simulink model "Target_Control_System"  (R2021b)
settings: Solver=FixedStepDiscrete  StartTime=0.0  StopTime=5  RelTol=1e-3
PreLoadFcn:
  | RTWConfigurationCB('preloadfcn', bdroot);
PostLoadFcn:
  | load('configuration/data_struct.mat');
  | load('configuration/fluxMaps_propMotor.mat');
  | load('configuration/parameterInit_PROP.mat');
  | load('configuration/parameterInit_PUMP.mat');
  | load('configuration/parameterInit_PITCH.mat');
  | load('configuration/parameterInit_TILT.mat');
  | %load('configuration/base_workspace_signal_definition.mat');
  | %load('resolvedatastores_to_baseworkspace_for_faster_simulation.mat');
model workspace (MAT data in the model file):
  SIMULATION_OPTIONS : Simulink.Parameter (value not decoded)
  TARGET_CODE_GEN : Simulink.Parameter (value not decoded)
  TCS_SAMPLE_FREQ_HZ : Simulink.Parameter (value not decoded)
symbols that are objects in the model workspace (value not decoded): TARGET_CODE_GEN, TCS_SAMPLE_FREQ_HZ
undefined symbols (not defined in the file): A_DQ_REF_LPF_INIT__PITCH, A_DQ_REF_LPF_INIT__PROP, A_DQ_REF_LPF_INIT__PUMP, A_DQ_REF_LPF_INIT__TILT, A_OBSERVER_CONFIDENCE_INIT__PITCH, A_OBSERVER_CONFIDENCE_INIT__PROP, A_OBSERVER_CONFIDENCE_INIT__PUMP, A_OBSERVER_CONFIDENCE_INIT__TILT, ACTUATOR_MAX_ANGLE_TRIP__PITCH, ACTUATOR_MIN_ANGLE_TRIP__PITCH, ACTUATOR_POS_SENSOR_INV_DIRECTION__PITCH, ACTUATOR_POS_SENSOR_INV_DIRECTION__TILT, ACTUATOR_POS_SENSOR_OFFSET__PITCH, ACTUATOR_POS_SENSOR_OFFSET__TILT, ADC_scaler1_baseaddr_TILT, ADC_SCALER_FLOAT_TO_FIXPOINT_EXPANSION, ANGLE_ELEC_FROM_SENSOR_OFFSET_INIT__PITCH, ANGLE_ELEC_FROM_SENSOR_OFFSET_INIT__PROP, ANGLE_ELEC_FROM_SENSOR_OFFSET_INIT__PUMP, ANGLE_ELEC_FROM_SENSOR_OFFSET_INIT__TILT, AUTO_CLEAR_FAULTS_ENABLED__PITCH, AUTO_CLEAR_FAULTS_ENABLED__PROP, AUTO_CLEAR_FAULTS_ENABLED__PUMP, AUTO_CLEAR_FAULTS_ENABLED__TILT, AUTO_CLEAR_FAULTS_WAIT_TICKS__PITCH, AUTO_CLEAR_FAULTS_WAIT_TICKS__PROP, AUTO_CLEAR_FAULTS_WAIT_TICKS__PUMP, AUTO_CLEAR_FAULTS_WAIT_TICKS__TILT, AUTO_I_ZERO_IDLE_TICKS__PITCH, AUTO_I_ZERO_IDLE_TICKS__PROP, AUTO_I_ZERO_IDLE_TICKS__PUMP, AUTO_I_ZERO_IDLE_TICKS__TILT, AUTO_I_ZERO_OFFSET_IDC_THRESHOLD__PITCH, AUTO_I_ZERO_OFFSET_IDC_THRESHOLD__PROP, AUTO_I_ZERO_OFFSET_IDC_THRESHOLD__PUMP, AUTO_I_ZERO_OFFSET_IDC_THRESHOLD__TILT, AUTO_I_ZERO_OFFSET_IPH_THRESHOLD__PITCH, AUTO_I_ZERO_OFFSET_IPH_THRESHOLD__PROP, AUTO_I_ZERO_OFFSET_IPH_THRESHOLD__PUMP, AUTO_I_ZERO_OFFSET_IPH_THRESHOLD__TILT, AUTO_SENSORLESS_SWITCHOVER_DISABLE_OMEGA, AUTO_SENSORLESS_SWITCHOVER_ENABLE_OMEGA, AUTO_SENSORLESS_SWITCHOVER_MIN_CONFIDENCE, AUXILIARY_PROTECTION_UNIT_BASEADDR__TILT, blanking_max_error_omega_INIT_PITCH, blanking_max_error_omega_INIT_TILT, blanking_max_error_position_INIT_PITCH, blanking_max_error_position_INIT_TILT, BRUTE_START_I_Q_REF_RAMP_SPEED__PITCH, BRUTE_START_I_Q_REF_RAMP_SPEED__PROP, BRUTE_START_I_Q_REF_RAMP_SPEED__PUMP, BRUTE_START_I_Q_REF_RAMP_SPEED__TILT, CONTROL_LOOP_DT_INIT__PITCH, CONTROL_LOOP_DT_INIT__PROP, CONTROL_LOOP_DT_INIT__PUMP, CONTROL_LOOP_DT_INIT__TILT, CORRECTION_FILTER_SCALE__PITCH, CORRECTION_FILTER_SCALE__PROP, CORRECTION_FILTER_SCALE__PUMP, CORRECTION_FILTER_SCALE__TILT ... (+458)
libraries: simulink x178, Reusables_Lib x24
(part 30 of 47)

== system Target_Control_System/Target_Control_System/MainLoop/tiltMotor_mainLoop/mainTask_tilt/motorTaskMainFastStep(&oTilt)/Control Loops - Tilt ==
  note: // Ramp Id, also include a fixed fraction of Iq (happens in the interupt)
  note: // Feed-forward of speed reference derivative into torque
      | // --- Would go here if needed --- (Blend the ramp generator ddt output into Iq ref)
  note: // Static current limiting only
  note: // The greater than 0 is needed to allow regen braking when the speed is high enough
  note: // Ramp position setpoint
  note: // Blend in the idle controller's contribution (don't add; disturbs Torque/Amp relation).
      | // Take the max of both, but only if the idle controller is active)
  note: // Ramp angle compensation value for smoothing of forced to closed loop operation
      |  // It always ramps to zero.
  note: // no feedforward in forced angle, because the speed estimate may be garbage
  controlLoops : TriggerPort  TriggerType=function-call  VariantControl=Variant
  AND1 : Logic  AllPortsSameDT=off  OutDataTypeStr=boolean
  Constant13 : Constant  Value=CONTROL_LOOP_DT_INIT__TILT  OutDataTypeStr=single  SampleTime=-1
  Constant2 : Constant  Commented=on  Value=0  SampleTime=-1
  Constant3 : Constant  Value=0  SampleTime=-1
  Constant4 : Constant  Value=0.001  OutDataTypeStr=single  SampleTime=-1
  Constant5 : Constant  Commented=on  Value=0  OutDataTypeStr=single  SampleTime=-1
  Constant6 : Constant  Value=0  OutDataTypeStr=single  SampleTime=-1
  Constant7 : Constant  Value=ISR_FREQ_KHZ__TILT  OutDataTypeStr=single  SampleTime=-1
  Data Store Read10 : DataStoreRead  DataStoreName=oTilt  DataStoreElements=oTilt.oMot_.oState_.oRampDataIdRef_.oParam_.fDownslope_  IndexOptions=Index vector (dialog)  Indices=1  OutputSizes=1
  Data Store Read104 : DataStoreRead  Commented=on  DataStoreName=oTilt  DataStoreElements=oTilt.oMot_.oOut_.uiForcedAngle_  IndexOptions=Index vector (dialog)  Indices=1  OutputSizes=1
  Data Store Read11 : DataStoreRead  DataStoreName=oTilt  DataStoreElements=oTilt.oMot_.oState_.oRampDataIdRef_.oParam_.fUpslope_  IndexOptions=Index vector (dialog)  Indices=1  OutputSizes=1
  Data Store Read110 : DataStoreRead  Commented=on  DataStoreName=oTilt  DataStoreElements=oTilt.oMot_.oState_.oRampDataFluxMstrAngFrcd2clsdSmoothn_.oParam_.fUpslope_  IndexOptions=Index vector (dialog)  Indices=1  OutputSizes=1
  Data Store Read111 : DataStoreRead  Commented=on  DataStoreName=oTilt  DataStoreElements=oTilt.oMot_.oState_.oRampDataFluxMstrAngFrcd2clsdSmoothn_.oParam_.fDownslope_  IndexOptions=Index vector (dialog)  Indices=1  OutputSizes=1
  Data Store Read112 : DataStoreRead  Commented=on  DataStoreName=oTilt  DataStoreElements=oTilt.oMot_.oState_.oRampDataFluxMstrAngFrcd2clsdSmoothn_.oParam_.fTimestepS_  IndexOptions=Index vector (dialog)  Indices=1  OutputSizes=1
  Data Store Read12 : DataStoreRead  DataStoreName=oTilt  DataStoreElements=oTilt.oMot_.oState_.oRampDataIdRef_.oParam_.fTimestepS_  IndexOptions=Index vector (dialog)  Indices=1  OutputSizes=1
  Data Store Read13 : DataStoreRead  DataStoreName=oTilt  DataStoreElements=oTilt.oMot_.oState_.oPosSensor_.iPosControlEnabled_  IndexOptions=Index vector (dialog)  Indices=1  OutputSizes=1
  Data Store Read14 : DataStoreRead  DataStoreName=oTilt  DataStoreElements=oTilt.oMot_.oState_.oRampDataOmegaERef_.fSetpoint_  IndexOptions=Index vector (dialog)  Indices=1  OutputSizes=1
  Data Store Read15 : DataStoreRead  DataStoreName=oTilt  DataStoreElements=oTilt.oMot_.oParam_.fDynILimIntegratorLeakageFactor_  IndexOptions=Index vector (dialog)  Indices=1  OutputSizes=1
  Data Store Read16 : DataStoreRead  DataStoreName=oTilt  DataStoreElements=oTilt.oMot_.oState_.fIdleCtrlCurrent_  IndexOptions=Index vector (dialog)  Indices=1  OutputSizes=1
  Data Store Read17 : DataStoreRead  DataStoreName=oTilt  DataStoreElements=oTilt.oMot_.oParam_.fIqSetpointMax_  IndexOptions=Index vector (dialog)  Indices=1  OutputSizes=1
  Data Store Read19 : DataStoreRead  DataStoreName=oTilt  DataStoreElements=oTilt.oMot_.oParam_.fPositionRefFfwdToOmega_  IndexOptions=Index vector (dialog)  Indices=1  OutputSizes=1
  Data Store Read2 : DataStoreRead  Commented=on  DataStoreName=oTilt  DataStoreElements=oTilt.oMot_.oState_.oRampDataFluxMasterAngleOffset_.fSetpoint_  IndexOptions=Index vector (dialog)  Indices=1  OutputSizes=1
  Data Store Read20 : DataStoreRead  DataStoreName=oTilt  DataStoreElements=oTilt.oMot_.oState_.oRampDataIqRef_.oParam_.fUpslope_  IndexOptions=Index vector (dialog)  Indices=1  OutputSizes=1
  Data Store Read21 : DataStoreRead  DataStoreName=oTilt  DataStoreElements=oTilt.oMot_.oState_.fIqRefBeforeRamp_  IndexOptions=Index vector (dialog)  Indices=1  OutputSizes=1
  Data Store Read22 : DataStoreRead  DataStoreName=oTilt  DataStoreElements=oTilt.oMot_.oState_.oRampDataIqRef_.oParam_.fDownslope_  IndexOptions=Index vector (dialog)  Indices=1  OutputSizes=1
  Data Store Read23 : DataStoreRead  Commented=on  DataStoreName=oTilt  DataStoreElements=oTilt.oMot_.oState_.oRampDataFluxFeedforwardGain_.fRampOut_  IndexOptions=Index vector (dialog)  Indices=1  OutputSizes=1
  Data Store Read27 : DataStoreRead  DataStoreName=oTilt  DataStoreElements=oTilt.oMot_.oState_.oRampDataOmegaERef_.oParam_.fUpslope_  IndexOptions=Index vector (dialog)  Indices=1  OutputSizes=1
  Data Store Read28 : DataStoreRead  DataStoreName=oTilt  DataStoreElements=oTilt.oMot_.oState_.uiSpeedControllerActive_  IndexOptions=Index vector (dialog)  Indices=1  OutputSizes=1
  Data Store Read29 : DataStoreRead  DataStoreName=oTilt  DataStoreElements=oTilt.oMot_.oState_.oRampDataOmegaERef_.oParam_.fTimestepS_  IndexOptions=Index vector (dialog)  Indices=1  OutputSizes=1
  Data Store Read3 : DataStoreRead  Commented=on  DataStoreName=oTilt  DataStoreElements=oTilt.oMot_.oState_.oRampDataFluxMasterAngleOffset_.oParam_.fUpslope_  IndexOptions=Index vector (dialog)  Indices=1  OutputSizes=1
  Data Store Read30 : DataStoreRead  DataStoreName=oTilt  DataStoreElements=oTilt.oMot_.oState_.oRampDataPos_.oParam_.fUpslope_  IndexOptions=Index vector (dialog)  Indices=1  OutputSizes=1
  Data Store Read31 : DataStoreRead  DataStoreName=oTilt  DataStoreElements=oTilt.oMot_.oState_.oRampDataOmegaERef_.oParam_.fDownslope_  IndexOptions=Index vector (dialog)  Indices=1  OutputSizes=1
  Data Store Read32 : DataStoreRead  DataStoreName=oTilt  DataStoreElements=oTilt.oMot_.oState_.oRampDataPos_.oParam_.fDownslope_  IndexOptions=Index vector (dialog)  Indices=1  OutputSizes=1
  Data Store Read33 : DataStoreRead  DataStoreName=oTilt  DataStoreElements=oTilt.oMot_.oState_.oRampDataPos_.fSetpoint_  IndexOptions=Index vector (dialog)  Indices=1  OutputSizes=1
  Data Store Read4 : DataStoreRead  DataStoreName=oTilt  DataStoreElements=oTilt.oMot_.oState_.oRampDataIqRef_.oParam_.fTimestepS_  IndexOptions=Index vector (dialog)  Indices=1  OutputSizes=1
  Data Store Read5 : DataStoreRead  Commented=on  DataStoreName=oTilt  DataStoreElements=oTilt.oMot_.oState_.oRampDataFluxMasterAngleOffset_.oParam_.fDownslope_  IndexOptions=Index vector (dialog)  Indices=1  OutputSizes=1
  Data Store Read88 : DataStoreRead  Commented=on  DataStoreName=oTilt  DataStoreElements=oTilt.oMot_.oState_.oRampDataFluxMasterAngleOffset_.oParam_.fTimestepS_  IndexOptions=Index vector (dialog)  Indices=1  OutputSizes=1
  Data Store Write1 : DataStoreWrite  Commented=on  DataStoreName=oTilt  DataStoreElements=oTilt.oMot_.oState_.oRampDataFluxMstrAngFrcd2clsdSmoothn_.fSetpoint_  IndexOptions=Index vector (dialog)  Indices=1  OutputSizes=1
  Data Store Write10 : DataStoreWrite  DataStoreName=oTilt  DataStoreElements=oTilt.oMot_.oState_.oRampDataIdRef_.fRampOut_  IndexOptions=Index vector (dialog)  Indices=1  OutputSizes=1
  Data Store Write14 : DataStoreWrite  DataStoreName=oTilt  DataStoreElements=oTilt.oMot_.oState_.oRampDataIdRef_.fRampOutDdt_  IndexOptions=Index vector (dialog)  Indices=1  OutputSizes=1
  Data Store Write16 : DataStoreWrite  DataStoreName=oTilt  DataStoreElements=oTilt.oMot_.oState_.oRampDataOmegaERef_.fRampOutDdt_  IndexOptions=Index vector (dialog)  Indices=1  OutputSizes=1
  Data Store Write17 : DataStoreWrite  DataStoreName=oTilt  DataStoreElements=oTilt.oMot_.oState_.oRampDataOmegaERef_.fRampOut_  IndexOptions=Index vector (dialog)  Indices=1  OutputSizes=1
  Data Store Write18 : DataStoreWrite  DataStoreName=oTilt  DataStoreElements=oTilt.oMot_.oState_.oRampDataPos_.fRampOut_  IndexOptions=Index vector (dialog)  Indices=1  OutputSizes=1
  Data Store Write19 : DataStoreWrite  DataStoreName=oTilt  DataStoreElements=oTilt.oMot_.oState_.oRampDataPos_.fRampOutDdt_  IndexOptions=Index vector (dialog)  Indices=1  OutputSizes=1
  Data Store Write2 : DataStoreWrite  Commented=on  DataStoreName=oTilt  DataStoreElements=oTilt.oMot_.oState_.oRampDataFluxMasterAngleOffset_.fRampOut_  IndexOptions=Index vector (dialog)  Indices=1  OutputSizes=1
  Data Store Write3 : DataStoreWrite  Commented=on  DataStoreName=oTilt  DataStoreElements=oTilt.oMot_.oState_.oRampDataFluxMasterAngleOffset_.fRampOutDdt_  IndexOptions=Index vector (dialog)  Indices=1  OutputSizes=1
  Data Store Write4 : DataStoreWrite  DataStoreName=oTilt  DataStoreElements=oTilt.oMot_.oState_.oRampDataOmegaERef_.fSetpoint_  IndexOptions=Index vector (dialog)  Indices=1  OutputSizes=1
  Data Store Write5 : DataStoreWrite  DataStoreName=oTilt  DataStoreElements=oTilt.oMot_.oState_.oRampDataIqRef_.fRampOut_  IndexOptions=Index vector (dialog)  Indices=1  OutputSizes=1
  Data Store Write6 : DataStoreWrite  DataStoreName=oTilt  DataStoreElements=oTilt.oMot_.oState_.oRampDataIdRef_.fSetpoint_  IndexOptions=Index vector (dialog)  Indices=1  OutputSizes=1
  Data Store Write64 : DataStoreWrite  Commented=on  DataStoreName=oTilt  DataStoreElements=oTilt.oMot_.oState_.oRampDataFluxMstrAngFrcd2clsdSmoothn_.fRampOut_  IndexOptions=Index vector (dialog)  Indices=1  OutputSizes=1
  Data Store Write65 : DataStoreWrite  Commented=on  DataStoreName=oTilt  DataStoreElements=oTilt.oMot_.oState_.oRampDataFluxMstrAngFrcd2clsdSmoothn_.fRampOutDdt_  IndexOptions=Index vector (dialog)  Indices=1  OutputSizes=1
  Data Store Write66 : DataStoreWrite  Commented=on  DataStoreName=oTilt  DataStoreElements=oTilt.oMot_.oState_.oRampDataFluxFeedforwardGain_.fRampOut_  IndexOptions=Index vector (dialog)  Indices=1  OutputSizes=1
  Data Store Write7 : DataStoreWrite  DataStoreName=oTilt  DataStoreElements=oTilt.oMot_.oState_.oRampDataIqRef_.fRampOutDdt_  IndexOptions=Index vector (dialog)  Indices=1  OutputSizes=1
  Data Store Write8 : DataStoreWrite  DataStoreName=oTilt  DataStoreElements=oTilt.oMot_.oState_.oRampDataIqRef_.fSetpoint_  IndexOptions=Index vector (dialog)  Indices=1  OutputSizes=1
  Divide1 : Product  Inputs=**
  Dynamic Current Limiting Tilt : Subsystem  TreatAsAtomicUnit=on
  Flux Weakening Tilt : Subsystem
  Gain2 : Gain  Gain=-1
  GreaterThan4 : RelationalOperator  Commented=on  Operator=>  OutDataTypeStr=boolean  RndMeth=Simplest
  GreaterThan5 : RelationalOperator  Operator=>  OutDataTypeStr=boolean  RndMeth=Simplest
  GreaterThan6 : RelationalOperator  Operator=>  OutDataTypeStr=boolean  RndMeth=Simplest
  GreaterThan7 : RelationalOperator  Operator=>  OutDataTypeStr=boolean  RndMeth=Simplest
  Max2 : MinMax  Function=max  Inputs=2
  Min1 : MinMax  Inputs=2
  NOT : Logic  Commented=on  Operator=NOT  AllPortsSameDT=off  OutDataTypeStr=boolean
  Position Controller Tilt : Subsystem  TreatAsAtomicUnit=on
  Ramp Flux Feedforward : Subsystem  Commented=on  TreatAsAtomicUnit=on
  Speed Controller Tilt : Subsystem  TreatAsAtomicUnit=on
  Sum1 : Sum  Inputs=|++
  Switch1 : Switch  Criteria=u2 > Threshold
  Switch2 : Switch  Criteria=u2 > Threshold
  Switch3 : Switch  Criteria=u2 > Threshold
  Switch4 : Switch  Commented=on  Criteria=u2 > Threshold
  Unit Delay1 : UnitDelay  SampleTime=-1  HasFrameUpgradeWarning=on
  Zero11 : Constant  Commented=on  Value=0  OutDataTypeStr=single  SampleTime=-1
  pp_tilt : Gain  Gain=POLE_PAIRS_INIT__TILT  ParamDataTypeStr=single
  rampStep(oRampDataFluxMstrAngFrcd2clsdSmoothn)_tilt : Reusables_Lib/rampStep_  Commented=on  SystemSampleTime=-1  VariantActivationTime=update diagram  Latency=0  AutoFrameSizeCalculation=off
  rampStep(oRampDataPos)1 : Reusables_Lib/rampStep(oRampDataPos)  SystemSampleTime=-1  VariantActivationTime=update diagram  Latency=0  AutoFrameSizeCalculation=off
  rampStep_oRampDataFluxMasterAngleOffset_tilt : Reusables_Lib/rampStep_  Commented=on  SystemSampleTime=-1  VariantActivationTime=update diagram  Latency=0  AutoFrameSizeCalculation=off
  rampStep_oRampDataIdRef_ : Reusables_Lib/rampStep_  SystemSampleTime=-1  VariantActivationTime=update diagram  Latency=0  AutoFrameSizeCalculation=off
  rampStep_oRampDataIqRef_ : Reusables_Lib/rampStep_  SystemSampleTime=-1  VariantActivationTime=update diagram  Latency=0  AutoFrameSizeCalculation=off
  rampStep_oRampDataOmegaERef_ : Reusables_Lib/rampStep_  SystemSampleTime=-1  VariantActivationTime=update diagram  Latency=0  AutoFrameSizeCalculation=off
  to_CTRL_Hz1 : Gain  Gain=2*1000  ParamDataTypeStr=single  OutDataTypeStr=single
  wires:
  rampStep_oRampDataOmegaERef_/2 -> Data Store Write16/1
  rampStep_oRampDataIdRef_/2 -> Data Store Write14/1
  rampStep_oRampDataIdRef_/1 -> Data Store Write10/1
  rampStep_oRampDataFluxMasterAngleOffset_tilt/2 -> Data Store Write3/1
  rampStep_oRampDataFluxMasterAngleOffset_tilt/1 -> Data Store Write2/1
  rampStep(oRampDataFluxMstrAngFrcd2clsdSmoothn)_tilt/2 -> Data Store Write65/1
  rampStep(oRampDataFluxMstrAngFrcd2clsdSmoothn)_tilt/1 -> Data Store Write64/1
  Switch4/1 -> Data Store Write66/1
  Data Store Read5/1 -> rampStep_oRampDataFluxMasterAngleOffset_tilt/3
  Data Store Read2/1 -> rampStep_oRampDataFluxMasterAngleOffset_tilt/1
  Data Store Read3/1 -> rampStep_oRampDataFluxMasterAngleOffset_tilt/2
  Data Store Read88/1 -> rampStep_oRampDataFluxMasterAngleOffset_tilt/4
  rampStep(oRampDataPos)1/2 -> pp_tilt/1, Data Store Write19/1
  Data Store Read32/1 -> rampStep(oRampDataPos)1/4
  Data Store Read30/1 -> rampStep(oRampDataPos)1/3
  Data Store Read13/1 -> Position Controller Tilt/Enable, Switch2/2
  Data Store Read28/1 -> Speed Controller Tilt/Enable
  Data Store Read14/1 -> Switch2/3
  Switch2/1 -> Sum1/2
  rampStep_oRampDataOmegaERef_/1 -> Speed Controller Tilt/1(oRampDataOmegaERef_.fRampOut), Data Store Write17/1
  Data Store Read19/1 -> Divide1/2
  Constant7/1 -> to_CTRL_Hz1/1
  Data Store Read29/1 -> rampStep_oRampDataOmegaERef_/4
  Sum1/1 -> rampStep_oRampDataOmegaERef_/1, Data Store Write4/1
  Divide1/1 -> Sum1/1
  Data Store Read27/1 -> rampStep_oRampDataOmegaERef_/2
  Data Store Read31/1 -> rampStep_oRampDataOmegaERef_/3
  Data Store Read33/1 -> rampStep(oRampDataPos)1/1
  pp_tilt/1 -> Divide1/1
  Constant13/1 -> rampStep(oRampDataPos)1/6
  rampStep(oRampDataPos)1/1 -> Data Store Write18/1, Position Controller Tilt/1(oRampDataPos_.fRampOut), Unit Delay1/1
  Position Controller Tilt/1(oRampDataOmegaERef_.fSetpoint) -> Switch2/1
  to_CTRL_Hz1/1 -> rampStep(oRampDataPos)1/5
  Unit Delay1/1 -> rampStep(oRampDataPos)1/2
  Data Store Read11/1 -> rampStep_oRampDataIdRef_/2
  Flux Weakening Tilt/1(oRampDataIdRef_.fSetpoint) -> Data Store Write6/1, rampStep_oRampDataIdRef_/1
  Data Store Read10/1 -> rampStep_oRampDataIdRef_/3
  Data Store Read12/1 -> rampStep_oRampDataIdRef_/4
  Data Store Read20/1 -> rampStep_oRampDataIqRef_/2
  Data Store Read21/1 -> Min1/1
  Dynamic Current Limiting Tilt/1(oRampDataIqRef_.fSetpoint) -> Switch3/1
  Constant4/1 -> GreaterThan5/2
  rampStep_oRampDataIqRef_/1 -> Data Store Write5/1
  Switch3/1 -> GreaterThan6/2, Switch1/3
  rampStep_oRampDataIqRef_/2 -> Data Store Write7/1
  GreaterThan5/1 -> AND1/1
  Data Store Read17/1 -> Gain2/1, Min1/2
  Data Store Read22/1 -> rampStep_oRampDataIqRef_/3
  Switch1/1 -> Data Store Write8/1, rampStep_oRampDataIqRef_/1
  Data Store Read16/1 -> Switch1/1, GreaterThan6/1, GreaterThan5/1
  Min1/1 -> Max2/1
  GreaterThan7/1 -> Dynamic Current Limiting Tilt/Enable
  GreaterThan6/1 -> AND1/2
  Constant6/1 -> Switch3/2
  Max2/1 -> Switch3/3
  Data Store Read4/1 -> rampStep_oRampDataIqRef_/4
  Constant3/1 -> GreaterThan7/2
  AND1/1 -> Switch1/2
  Data Store Read15/1 -> GreaterThan7/1
  Gain2/1 -> Max2/2
  Data Store Read112/1 -> rampStep(oRampDataFluxMstrAngFrcd2clsdSmoothn)_tilt/4
  Constant5/1 -> Switch4/1
  Data Store Read111/1 -> rampStep(oRampDataFluxMstrAngFrcd2clsdSmoothn)_tilt/3
  NOT/1 -> Ramp Flux Feedforward/Enable
  GreaterThan4/1 -> NOT/1, Switch4/2
  Constant2/1 -> GreaterThan4/2
  Zero11/1 -> rampStep(oRampDataFluxMstrAngFrcd2clsdSmoothn)_tilt/1, Data Store Write1/1
  Data Store Read110/1 -> rampStep(oRampDataFluxMstrAngFrcd2clsdSmoothn)_tilt/2
  Data Store Read23/1 -> Switch4/3
  Data Store Read104/1 -> GreaterThan4/1

== system Target_Control_System/Target_Control_System/MainLoop/tiltMotor_mainLoop/mainTask_tilt/motorTaskMainFastStep(&oTilt)/Correction Constants for Observer and Control - Tilt ==
  note: // --- Angle and amplitude correction of the digital IIR filter ---
      | // First, we need to know the speed:
  note: // But forced angle overrules everything
  note: // Convert delay to angle
  note: // Now compute 1.a + 2.a:
  note: // Make the sign match the rotational direction
  note: // Add delay 3:
  note: // delay, in seconds (but the typical value will be under 100-200 us)
  note: // Delay (positive number) = np.arctan2(np.sqrt(2)*opStates->fOmegaRel_, (1-opStates->fOmegaRel_**2))
  note: // This is delay 1.b.2 MvdG: Ponder about the sign
  note: // Analytically calculate FPGA IIR filter characteristics (delay 1.b.2)
      |  // G =  1/np.sqrt(1+(fOmegaE/omega_e_3dB)**4)
  note: // Add delay 1.b.1
  note: // ---------------- Correction constants for observer and control ------------
      | // Sources of delay:
      | // 1. Input.
      | // a) delays from ADCs. Both voltage and current channels use identical ADCs and
      | // initial FPGA processing. The delay on the current channel is taken as a
      | // baseline.
      | //
      | // b) Extra delays in the voltage acquisition stage, due to
      | // 1) tighter analog filtering
      | // 2) the 2 pole LPF filter in the FPGA.
      | //
      | // 2. Output
      | // a) The PWM duty is updated only once per cycle, causing some delay.
      | // Additionally, the interrupt might be delayed, causing further delays.
      | //
      | // 3. User specified for testing
      | //
      | // Values of the above delays:
      | // 1.a A known constant delay is specified for each motor channel. (Mostly driven by the sinc3 filtering.
      | // Directly depends on sigma delta frequency.)
      | // 1.b.1 A known constant delay is specified for each motor channel
      | // 1.b.2 Can be calculated analytically
      | // 2.a Approximated as a constant fraction of the PWM period.
      | //
      | // Compensation order of the above delays
      | // - The entire interrupt loop runs behind reality by amount 1.a
      | // - The delay on the current acquisition is therefore not compensated at the input to the algorithm.
      | // - The voltage feedback needs to be aligned with the current feedback, and therefore needs to be
      | // corrected for delays 1.b.1 and 1.b.2. This is a phase shift applied to the voltage.
      | // - After the control loop, when the dq quantities are transformed to abc, the remaining delays are
      | // corrected by phase shifting the dq angle. These delays are 1.a, 2.a and 3.
      | //
      | // Additionally, filter 1.b.2 causes a reduction in amplitude. This is compensated too to ensure
      | // a more level flux estimate output at high speeds.
      | //
  correctionConstantsObserverControl : TriggerPort  TriggerType=function-call  VariantControl=Variant
  1/sqrt(1+u^2)1 : Subsystem
  Abs1 : Abs
  Abs2 : Abs  OutDataTypeStr=single
  Abs3 : Abs
  Add16 : Sum  Inputs=|++
  Add17 : Sum  Inputs=-+
  Atan2 : Trigonometry  Operator=atan2
  Constant29 : Constant  OutDataTypeStr=single  SampleTime=-1
  Data Store Read103 : DataStoreRead  DataStoreName=oTilt  DataStoreElements=oTilt.oMot_.oParam_.fFluxMasterAngleOffsetUser_  IndexOptions=Index vector (dialog)  Indices=1  OutputSizes=1
  Data Store Read2 : DataStoreRead  DataStoreName=oTilt  DataStoreElements=oTilt.oMot_.oState_.oRampDataOmegaERef_.fRampOut_  IndexOptions=Index vector (dialog)  Indices=1  OutputSizes=1
  Data Store Read3 : DataStoreRead  DataStoreName=oTilt  DataStoreElements=oTilt.oIsr_.oParam_.iUseSensorAngle_  IndexOptions=Index vector (dialog)  Indices=1  OutputSizes=1
  Data Store Read4 : DataStoreRead  DataStoreName=oTilt  DataStoreElements=oTilt.oMot_.oOut_.uiForcedAngle_  IndexOptions=Index vector (dialog)  Indices=1  OutputSizes=1
  Data Store Read5 : DataStoreRead  DataStoreName=oTilt  DataStoreElements=oTilt.oMot_.oState_.oPosSensor_.fOmegaEFromSensor_  IndexOptions=Index vector (dialog)  Indices=1  OutputSizes=1
  Data Store Read6 : DataStoreRead  DataStoreName=oTilt  DataStoreElements=oTilt.oMot_.oIn_.fOmegaEObserverLpf2_  IndexOptions=Index vector (dialog)  Indices=1  OutputSizes=1
  Data Store Read92 : DataStoreRead  DataStoreName=oTilt  DataStoreElements=oTilt.oMot_.oParam_.fHardwareDelayCurrentAcquisition_  IndexOptions=Index vector (dialog)  Indices=1  OutputSizes=1
  Data Store Read93 : DataStoreRead  DataStoreName=oTilt  DataStoreElements=oTilt.oMot_.oParam_.fIntControlLoopDt_  IndexOptions=Index vector (dialog)  Indices=1  OutputSizes=1
  Data Store Read95 : DataStoreRead  DataStoreName=oTilt  DataStoreElements=oTilt.oMot_.oParam_.fUphaseIirFLpfRads_  IndexOptions=Index vector (dialog)  Indices=1  OutputSizes=1
  Data Store Read97 : DataStoreRead  DataStoreName=oTilt  DataStoreElements=oTilt.oMot_.oParam_.fHardwareDelayVoltageAcquisitionExtra_  IndexOptions=Index vector (dialog)  Indices=1  OutputSizes=1
  Data Store Read99 : DataStoreRead  DataStoreName=oTilt  DataStoreElements=oTilt.oMot_.oParam_.fHardwareDelayControlLoopFraction_  IndexOptions=Index vector (dialog)  Indices=1  OutputSizes=1
  Data Store Write1 : DataStoreWrite  DataStoreName=mdl_tilt_fOmegaE  IndexOptions=Index vector (dialog)  Indices=1  OutputSizes=1
  Data Store Write40 : DataStoreWrite  DataStoreName=oTilt  DataStoreElements=oTilt.oMot_.oState_.oRampDataFluxMasterAngleOffset_.fSetpoint_  IndexOptions=Index vector (dialog)  Indices=1  OutputSizes=1
  Data Store Write41 : DataStoreWrite  DataStoreName=oTilt  DataStoreElements=oTilt.oMot_.oState_.fOmegaRel_  IndexOptions=Index vector (dialog)  Indices=1  OutputSizes=1
  Data Store Write43 : DataStoreWrite  DataStoreName=oTilt  DataStoreElements=oTilt.oMot_.oOut_.fUphFilterAmplitudeRatio_  IndexOptions=Index vector (dialog)  Indices=1  OutputSizes=1
  Data Store Write44 : DataStoreWrite  DataStoreName=oTilt  DataStoreElements=oTilt.oMot_.oOut_.fUphFilterDelayAngleRad_  IndexOptions=Index vector (dialog)  Indices=1  OutputSizes=1
  Divide1 : Product  Inputs=/*
  Divide{3,8..9,21} (4 alike) : Product  Inputs=**
  Gain2 : Gain  Gain=sqrt(2)
  Product3 : Product
  Product4 : Product
  Saturation1 : Saturate  UpperLimit=inf  LowerLimit=0.3
  Saturation2 : Saturate  UpperLimit=pi/2  LowerLimit=-inf
  Sign1 : Signum
  Sign4 : Signum
  Sum3 : Sum  Inputs=|++
  Sum4 : Sum  Inputs=|++
  Switch1 : Switch  Criteria=u2 > Threshold
  Switch2 : Switch  Criteria=u2 > Threshold
  wires:
  Data Store Read2/1 -> Switch2/1
  Switch1/1 -> Switch2/3
  Data Store Read5/1 -> Switch1/1
  Data Store Read3/1 -> Switch1/2
  Data Store Read6/1 -> Switch1/3
  Data Store Read4/1 -> Switch2/2
  Data Store Read95/1 -> Divide1/1
  Divide9/1 -> Sum4/1  "fHardwareDelayAngleRad"
  Data Store Read99/1 -> Divide8/2
  Sum4/1 -> Product4/2
  Abs3/1 -> Divide9/1
  Product4/1 -> Data Store Write40/1
  Divide8/1 -> Sum3/2
  Sum3/1 -> Divide9/2  "fTemp"
  Switch2/1 -> Abs1/1, Sign1/1, Abs3/1, Sign4/1, Data Store Write1/1
  Data Store Read103/1 -> Sum4/2
  Sign4/1 -> Product4/1
  Data Store Read93/1 -> Divide8/1
  Data Store Read92/1 -> Sum3/1
  Saturation1/1 -> Data Store Write43/1
  Add17/1 -> Atan2/2
  Divide1/1 -> Data Store Write41/1, Divide3/1, Divide3/2, Gain2/1
  Abs2/1 -> Divide21/1
  Product3/1 -> Add16/2
  Add16/1 -> Saturation2/1
  Constant29/1 -> Add17/2
  Atan2/1 -> Add16/1
  Abs1/1 -> Product3/1, Divide1/2
  Divide21/1 -> Data Store Write44/1
  Sign1/1 -> Divide21/2
  Saturation2/1 -> Abs2/1
  Data Store Read97/1 -> Product3/2
  Divide3/1 -> 1/sqrt(1+u^2)1/1(fTemp), Add17/1  "fTemp"
  Gain2/1 -> Atan2/1
  1/sqrt(1+u^2)1/1(Out1) -> Saturation1/1

== system Target_Control_System/Target_Control_System/MainLoop/tiltMotor_mainLoop/mainTask_tilt/motorTaskMainFastStep(&oTilt)/Lowpass Filtered Quantities for External World - Tilt ==
  lpfQuantities : TriggerPort  TriggerType=function-call  VariantControl=Variant
  Constant25 : Constant  Value=0.00008  OutDataTypeStr=single  SampleTime=-1
  Data Store Read29 : DataStoreRead  DataStoreName=oTilt  DataStoreElements=oTilt.oMot_.oState_.fIPhaseMagnitudeLpf_  IndexOptions=Index vector (dialog)  Indices=1  OutputSizes=1
  Data Store Read30 : DataStoreRead  DataStoreName=oTilt  DataStoreElements=oTilt.oMot_.oIn_.oAdcData_.fUdc_  IndexOptions=Index vector (dialog)  Indices=1  OutputSizes=1
  Data Store Read33 : DataStoreRead  DataStoreName=oTilt  DataStoreElements=oTilt.oMot_.oOut_.fUdcLpf_  IndexOptions=Index vector (dialog)  Indices=1  OutputSizes=1
  Data Store Read4 : DataStoreRead  DataStoreName=oTilt  DataStoreElements=oTilt.oMot_.oIn_.fId_  IndexOptions=Index vector (dialog)  Indices=1  OutputSizes=1
  Data Store Read47 : DataStoreRead  DataStoreName=oTilt  DataStoreElements=oTilt.oMot_.oIn_.oAdcData_.fIdc_  IndexOptions=Index vector (dialog)  Indices=1  OutputSizes=1
  Data Store Read48 : DataStoreRead  DataStoreName=oTilt  DataStoreElements=oTilt.oMot_.oOut_.fIdcLpf_  IndexOptions=Index vector (dialog)  Indices=1  OutputSizes=1
  Data Store Read49 : DataStoreRead  DataStoreName=oTilt  DataStoreElements=oTilt.oMot_.oIn_.fPowerDc_  IndexOptions=Index vector (dialog)  Indices=1  OutputSizes=1
  Data Store Read5 : DataStoreRead  DataStoreName=oTilt  DataStoreElements=oTilt.oMot_.oIn_.fIq_  IndexOptions=Index vector (dialog)  Indices=1  OutputSizes=1
  Data Store Read50 : DataStoreRead  DataStoreName=oTilt  DataStoreElements=oTilt.oMot_.oOut_.fPowerDcLpf_  IndexOptions=Index vector (dialog)  Indices=1  OutputSizes=1
  Data Store Read51 : DataStoreRead  DataStoreName=oTilt  DataStoreElements=oTilt.oMot_.oIn_.fTEstimate_  IndexOptions=Index vector (dialog)  Indices=1  OutputSizes=1
  Data Store Read52 : DataStoreRead  DataStoreName=oTilt  DataStoreElements=oTilt.oMot_.oOut_.fTEstimateLpf_  IndexOptions=Index vector (dialog)  Indices=1  OutputSizes=1
  Data Store Read53 : DataStoreRead  DataStoreName=oTilt  DataStoreElements=oTilt.oMot_.oState_.oRampDataIqRef_.fRampOut_  IndexOptions=Index vector (dialog)  Indices=1  OutputSizes=1
  Data Store Read54 : DataStoreRead  DataStoreName=oTilt  DataStoreElements=oTilt.oMot_.oOut_.fIqRefRampOutLpf_  IndexOptions=Index vector (dialog)  Indices=1  OutputSizes=1
  Data Store Read55 : DataStoreRead  DataStoreName=oTilt  DataStoreElements=oTilt.oMot_.oParam_.fADqRefLpf_  IndexOptions=Index vector (dialog)  Indices=1  OutputSizes=1
  Data Store Read56 : DataStoreRead  DataStoreName=oTilt  DataStoreElements=oTilt.oMot_.oIn_.fIdRefTotal_  IndexOptions=Index vector (dialog)  Indices=1  OutputSizes=1
  Data Store Read57 : DataStoreRead  DataStoreName=oTilt  DataStoreElements=oTilt.oMot_.oOut_.fIdRefLpf_  IndexOptions=Index vector (dialog)  Indices=1  OutputSizes=1
  Data Store Read58 : DataStoreRead  DataStoreName=oTilt  DataStoreElements=oTilt.oMot_.oIn_.fUqRef_  IndexOptions=Index vector (dialog)  Indices=1  OutputSizes=1
  Data Store Read59 : DataStoreRead  DataStoreName=oTilt  DataStoreElements=oTilt.oMot_.oOut_.fUqRefLpf_  IndexOptions=Index vector (dialog)  Indices=1  OutputSizes=1
  Data Store Read6 : DataStoreRead  DataStoreName=oTilt  DataStoreElements=oTilt.oMot_.oOut_.fIdLpf_  IndexOptions=Index vector (dialog)  Indices=1  OutputSizes=1
  Data Store Read60 : DataStoreRead  DataStoreName=oTilt  DataStoreElements=oTilt.oMot_.oIn_.fUdRef_  IndexOptions=Index vector (dialog)  Indices=1  OutputSizes=1
  Data Store Read62 : DataStoreRead  DataStoreName=oTilt  DataStoreElements=oTilt.oMot_.oOut_.fUdRefLpf_  IndexOptions=Index vector (dialog)  Indices=1  OutputSizes=1
  Data Store Read63 : DataStoreRead  DataStoreName=oTilt  DataStoreElements=oTilt.oMot_.oOut_.fPowerDcLpf_  IndexOptions=Index vector (dialog)  Indices=1  OutputSizes=1
  Data Store Read64 : DataStoreRead  DataStoreName=oTilt  DataStoreElements=oTilt.oMot_.oOut_.fPowerDcXlpf_  IndexOptions=Index vector (dialog)  Indices=1  OutputSizes=1
  Data Store Read65 : DataStoreRead  DataStoreName=oTilt  DataStoreElements=oTilt.oMot_.oIn_.fOmegaEObserverLpf2_  IndexOptions=Index vector (dialog)  Indices=1  OutputSizes=1
  Data Store Read66 : DataStoreRead  DataStoreName=oTilt  DataStoreElements=oTilt.oMot_.oOut_.fOmegaEObserverXlpf2_  IndexOptions=Index vector (dialog)  Indices=1  OutputSizes=1
  Data Store Read69 : DataStoreRead  DataStoreName=oTilt  DataStoreElements=oTilt.oMot_.oParam_.fAOmegaXfilter2_  IndexOptions=Index vector (dialog)  Indices=1  OutputSizes=1
  Data Store Read7 : DataStoreRead  DataStoreName=oTilt  DataStoreElements=oTilt.oMot_.oOut_.fIqLpf_  IndexOptions=Index vector (dialog)  Indices=1  OutputSizes=1
  Data Store Read8 : DataStoreRead  DataStoreName=oTilt  DataStoreElements=oTilt.oMot_.oParam_.fSlowPassFactor_  IndexOptions=Index vector (dialog)  Indices=1  OutputSizes=1
  Data Store Read9 : DataStoreRead  DataStoreName=oTilt  DataStoreElements=oTilt.oMot_.oIn_.fIPhaseMagnitude_  IndexOptions=Index vector (dialog)  Indices=1  OutputSizes=1
  Data Store Write20 : DataStoreWrite  DataStoreName=oTilt  DataStoreElements=oTilt.oMot_.oState_.fIPhaseMagnitudeLpf_  IndexOptions=Index vector (dialog)  Indices=1  OutputSizes=1
  Data Store Write21 : DataStoreWrite  DataStoreName=oTilt  DataStoreElements=oTilt.oMot_.oOut_.fIdLpf_  IndexOptions=Index vector (dialog)  Indices=1  OutputSizes=1
  Data Store Write22 : DataStoreWrite  DataStoreName=oTilt  DataStoreElements=oTilt.oMot_.oOut_.fIqLpf_  IndexOptions=Index vector (dialog)  Indices=1  OutputSizes=1
  Data Store Write24 : DataStoreWrite  DataStoreName=oTilt  DataStoreElements=oTilt.oMot_.oOut_.fUdcLpf_  IndexOptions=Index vector (dialog)  Indices=1  OutputSizes=1
  Data Store Write25 : DataStoreWrite  DataStoreName=oTilt  DataStoreElements=oTilt.oMot_.oOut_.fIdcLpf_  IndexOptions=Index vector (dialog)  Indices=1  OutputSizes=1
  Data Store Write28 : DataStoreWrite  DataStoreName=oTilt  DataStoreElements=oTilt.oMot_.oOut_.fPowerDcLpf_  IndexOptions=Index vector (dialog)  Indices=1  OutputSizes=1
  Data Store Write29 : DataStoreWrite  DataStoreName=oTilt  DataStoreElements=oTilt.oMot_.oOut_.fTEstimateLpf_  IndexOptions=Index vector (dialog)  Indices=1  OutputSizes=1
  Data Store Write30 : DataStoreWrite  DataStoreName=oTilt  DataStoreElements=oTilt.oMot_.oOut_.fIqRefRampOutLpf_  IndexOptions=Index vector (dialog)  Indices=1  OutputSizes=1
  Data Store Write31 : DataStoreWrite  DataStoreName=oTilt  DataStoreElements=oTilt.oMot_.oOut_.fIdRefLpf_  IndexOptions=Index vector (dialog)  Indices=1  OutputSizes=1
  Data Store Write32 : DataStoreWrite  DataStoreName=oTilt  DataStoreElements=oTilt.oMot_.oOut_.fUqRefLpf_  IndexOptions=Index vector (dialog)  Indices=1  OutputSizes=1
  Data Store Write34 : DataStoreWrite  DataStoreName=oTilt  DataStoreElements=oTilt.oMot_.oOut_.fUdRefLpf_  IndexOptions=Index vector (dialog)  Indices=1  OutputSizes=1
  Data Store Write35 : DataStoreWrite  DataStoreName=oTilt  DataStoreElements=oTilt.oMot_.oOut_.fPowerDcXlpf_  IndexOptions=Index vector (dialog)  Indices=1  OutputSizes=1
  Data Store Write36 : DataStoreWrite  DataStoreName=oTilt  DataStoreElements=oTilt.oMot_.oOut_.fOmegaEObserverXlpf2_  IndexOptions=Index vector (dialog)  Indices=1  OutputSizes=1
  Divide{8..20} (13 alike) : Product  Inputs=**
  Sum{4..5,7,10..11,13,15,18,20..22,25,29} (13 alike) : Sum  Inputs=|+-
  Sum{3,6,8..9,12,14,16..17,19,24,26,30..31} (13 alike) : Sum  Inputs=|++
  wires:
  Sum6/1 -> Data Store Write21/1
  Data Store Read6/1 -> Sum4/2, Sum6/2
  Sum3/1 -> Data Store Write20/1
  Data Store Read9/1 -> Sum7/1
  Data Store Read51/1 -> Sum15/1
  Data Store Read30/1 -> Sum13/1
  Data Store Read49/1 -> Sum11/1
  Data Store Read50/1 -> Sum14/2, Sum11/2
  Data Store Read56/1 -> Sum20/1
  Data Store Read4/1 -> Sum4/1
  Data Store Read60/1 -> Sum25/1
  Data Store Read58/1 -> Sum29/1
  Sum17/1 -> Data Store Write30/1
  Data Store Read33/1 -> Sum13/2, Sum9/2
  Sum12/1 -> Data Store Write25/1
  Sum25/1 -> Divide19/2
  Data Store Read65/1 -> Sum22/1
  Data Store Read54/1 -> Sum18/2, Sum17/2
  Sum29/1 -> Divide17/2
  Divide11/1 -> Sum14/1
  Sum4/1 -> Divide9/2
  Divide12/1 -> Sum9/1
  Constant25/1 -> Divide20/1
  Divide19/1 -> Sum31/1
  Data Store Read7/1 -> Sum5/2, Sum8/2
  Sum10/1 -> Divide13/2
  Data Store Read55/1 -> Divide15/1, Divide16/1, Divide19/1, Divide17/1
  Data Store Read62/1 -> Sum25/2, Sum31/2
  Divide20/1 -> Sum24/1
  Sum15/1 -> Divide14/2
  Sum21/1 -> Divide20/2
  Sum8/1 -> Data Store Write22/1
  Data Store Read5/1 -> Sum5/1
  Data Store Read53/1 -> Sum18/1
  Divide16/1 -> Sum19/1
  Data Store Read29/1 -> Sum7/2, Sum3/2
  Data Store Read48/1 -> Sum12/2, Sum10/2
  Divide13/1 -> Sum12/1
  Sum11/1 -> Divide11/2
  Divide15/1 -> Sum17/1
  Data Store Read64/1 -> Sum24/2, Sum21/2
  Sum5/1 -> Divide10/2
  Divide10/1 -> Sum8/1
  Sum22/1 -> Divide18/2
  Divide14/1 -> Sum16/1
  Divide18/1 -> Sum26/1
  Sum14/1 -> Data Store Write28/1
  Data Store Read52/1 -> Sum15/2, Sum16/2
  Sum24/1 -> Data Store Write35/1
  Sum26/1 -> Data Store Write36/1
  Data Store Read57/1 -> Sum20/2, Sum19/2
  Data Store Read59/1 -> Sum29/2, Sum30/2
  Sum7/1 -> Divide8/2
  Divide8/1 -> Sum3/1
  Divide17/1 -> Sum30/1
  Data Store Read66/1 -> Sum26/2, Sum22/2
  Sum31/1 -> Data Store Write34/1
  Sum18/1 -> Divide15/2
  Sum20/1 -> Divide16/2
  Data Store Read63/1 -> Sum21/1
  Sum30/1 -> Data Store Write32/1
  Data Store Read8/1 -> Divide8/1, Divide9/1, Divide10/1, Divide12/1, Divide13/1, Divide14/1, Divide11/1
  Data Store Read47/1 -> Sum10/1
  Data Store Read69/1 -> Divide18/1
  Divide9/1 -> Sum6/1
  Sum9/1 -> Data Store Write24/1
  Sum19/1 -> Data Store Write31/1
  Sum13/1 -> Divide12/2
  Sum16/1 -> Data Store Write29/1

== system Target_Control_System/Target_Control_System/MainLoop/tiltMotor_mainLoop/mainTask_tilt/motorTaskMainFastStep(&oTilt)/Mechanical System - Tilt ==
  mechanicalSystem : TriggerPort  TriggerType=function-call  VariantControl=Variant
  Data Store Read : DataStoreRead  DataStoreName=oTilt  DataStoreElements=oTilt.oMot_.oState_.oPosSensor_.eInputPositionSensorType_  IndexOptions=Index vector (dialog)  Indices=1  OutputSizes=1
  Enumerated Constant1 : simulink/Sources/Enumerated Constant  OutDataTypeStr=Enum: EPositionSensor_t  Value=EPositionSensor_t.eNone  SampleTime=-1
  NotEqual : RelationalOperator  Operator=~=  OutDataTypeStr=boolean  RndMeth=Simplest
  processSensors(&oPitch) : Subsystem  TreatAsAtomicUnit=on
  wires:
  Enumerated Constant1/1 -> NotEqual/2
  NotEqual/1 -> processSensors(&oPitch)/Enable
  Data Store Read/1 -> NotEqual/1

== system Target_Control_System/Target_Control_System/MainLoop/tiltMotor_mainLoop/mainTask_tilt/motorTaskMainFastStep(&oTilt)/Motor Acceleration - Tilt ==
  note: // Compute the acceleration (derivative of the speed). It is computed simply from the 1-step difference,
      |    // but strongly low pass filtered to ultimately end up with a bandwidth less than 50-100 Hz.
      |    // A filter running at the typical control frequency (80 kHz for the prop) would have to be too steep, so
      |    // a multi-stage, dual sample rate approach is used: A first filter runs at full control rate, with a cut-
      |    // off frequency of some 1-2 kHz. A second filter runs at 5 kHz and brings the bandwidth down to less than
      |    // 50-100 Hz.
      |    // At this location in the code, the first filter stage is executed:
  motorAcceleration : TriggerPort  TriggerType=function-call  VariantControl=Variant
  First filter stage : Subsystem  TreatAsAtomicUnit=on
  Function-Call Generator : simulink/Ports & Subsystems/Function-Call Generator  sample_time=-1  numberOfIterations=1  DisallowWideOutput=off
  Function-Call Split10 : FunctionCallSplit  NumOutputPorts=2
  Speed step : Subsystem
  wires:
  Function-Call Generator/1 -> Function-Call Split10/1
  Function-Call Split10/1 -> First filter stage/Trigger
  Function-Call Split10/2 -> Speed step/Trigger

== system Target_Control_System/Target_Control_System/MainLoop/tiltMotor_mainLoop/mainTask_tilt/motorTaskMainFastStep(&oTilt)/Observer Confidence - Tilt ==
  note: // ideally zero,
      | // but can go up to inf
  note: // Three contributions, each adding 1/3 to give a value in range 0.0-1.0:
      | //  1. Magnitude of estimated flux relative to nominal flux (perhaps not for induction motors)
      | //  REMOVED (for the time being) 2. The relative noise on the magnitude of the estimated flux (relative noise=magnitude of derivative/HPF divided by average value)
      | //  3. The relative noise on the estimated speed
  note: // If greater than 125% off,
      | // keep at 125%
  note: // the 0.4 is 0.5/tempf_max
  note: // 1. magnitude of flux. Map to a 0-0.33 range
  note: // 3. noise on estimated omega
  note: // ideally zero,
      | // but can go up to inf
  note: // If greater than X% off,
      | // keep at X%
  observerConfidence : TriggerPort  TriggerType=function-call  VariantControl=Variant
  Abs1 : Abs  OutDataTypeStr=single
  Abs4 : Abs  OutDataTypeStr=single
  Abs6 : Abs  OutDataTypeStr=single
  Add1 : Sum  Inputs=|-+
  Add12 : Sum  Inputs=+-
  Add13 : Sum  Inputs=|+-
  Add14 : Sum  Inputs=|-+
  Add15 : Sum  Inputs=|-+
  Add3 : Sum
  Add4 : Sum  Inputs=++|
  Constant28 : Constant  OutDataTypeStr=single  SampleTime=-1
  Data Store Read2 : DataStoreRead  DataStoreName=oTilt  DataStoreElements=oTilt.oMot_.oParam_.fAObserverConfidence_  IndexOptions=Index vector (dialog)  Indices=1  OutputSizes=1
  Data Store Read75 : DataStoreRead  DataStoreName=oTilt  DataStoreElements=oTilt.oMot_.oOut_.fOmegaEObserverXlpf2_  IndexOptions=Index vector (dialog)  Indices=1  OutputSizes=1
  Data Store Read79 : DataStoreRead  DataStoreName=oTilt  DataStoreElements=oTilt.oMot_.oIn_.fFluxMainMagnitudeLpf_  IndexOptions=Index vector (dialog)  Indices=1  OutputSizes=1
  Data Store Read84 : DataStoreRead  DataStoreName=oTilt  DataStoreElements=oTilt.oIsr_.oState_.fOmegaEObserverRaw2_  IndexOptions=Index vector (dialog)  Indices=1  OutputSizes=1
  Data Store Read86 : DataStoreRead  DataStoreName=oTilt  DataStoreElements=oTilt.oMot_.oParam_.fMainFluxNominal_  IndexOptions=Index vector (dialog)  Indices=1  OutputSizes=1
  Data Store Write1 : DataStoreWrite  DataStoreName=oTilt  DataStoreElements=oTilt.oMot_.oState_.fObserverConfidence_  IndexOptions=Index vector (dialog)  Indices=1  OutputSizes=1
  Divide2 : Product  Inputs=*/
  Divide4 : Product  Inputs=*/
  Gain1 : Gain  Gain=0.83
  Gain2 : Gain  Gain=0.4
  Half1 : Constant  Value=0.5  OutDataTypeStr=single  SampleTime=-1
  Half3 : Constant  Value=0.5  OutDataTypeStr=single  SampleTime=-1
  IIR1 : Subsystem
  Saturation1 : Saturate  UpperLimit=1.25  LowerLimit=-inf
  Saturation4 : Saturate  UpperLimit=0.6  LowerLimit=-inf
  Sum23 : Sum  Inputs=-+|
  Switch18 : Switch  Criteria=u2 > Threshold  Threshold=0.5
  Unit Delay2 : UnitDelay  SampleTime=-1  HasFrameUpgradeWarning=on
  Zero1 : Constant  Value=0  OutDataTypeStr=Inherit: Inherit via back propagation  SampleTime=-1
  fAObserverConfidence_ : Gain  Gain=0.01
  isNaN1 : RelationalOperator  Operator=isNaN  OutDataTypeStr=boolean  RndMeth=Simplest
  wires:
  Divide4/1 -> Saturation4/1
  Abs6/1 -> Divide4/2
  Data Store Read84/1 -> Add15/1
  Half1/1 -> Add14/2
  Add1/1 -> Add3/2
  Data Store Read2/1 -> IIR1/3(K), Add12/2
  Add3/1 -> isNaN1/1, Switch18/3  "fObserverConfidenceRaw_"
  Zero1/1 -> Switch18/1
  Saturation4/1 -> Gain1/1
  Divide2/1 -> Saturation1/1
  Add13/1 -> Abs1/1
  fAObserverConfidence_/1 -> Add4/2
  Unit Delay2/1 -> Sum23/1, Add4/1
  IIR1/1(Out) -> Data Store Write1/1
  Sum23/1 -> fAObserverConfidence_/1
  Data Store Read86/1 -> Add13/2, Divide2/2
  Abs1/1 -> Divide2/1
  Add15/1 -> Abs4/1
  Constant28/1 -> Add12/1
  isNaN1/1 -> Switch18/2
  Switch18/1 -> Sum23/2, IIR1/1(In)
  Data Store Read79/1 -> Add13/1
  Gain1/1 -> Add1/1
  Data Store Read75/1 -> Abs6/1, Add15/2
  Add4/1 -> Unit Delay2/1
  Abs4/1 -> Divide4/1
  Add14/1 -> Add3/1
  Saturation1/1 -> Gain2/1
  Add12/1 -> IIR1/2(1-K)
  Gain2/1 -> Add14/1
  Half3/1 -> Add1/2

== system Target_Control_System/Target_Control_System/MainLoop/tiltMotor_mainLoop/mainTask_tilt/motorTaskMainFastStep(&oTilt)/Software Overcurrent Protection - Tilt ==
  overcurrentProtection : TriggerPort  TriggerType=function-call  VariantControl=Variant
  Constant7 : Constant  Value=211  OutDataTypeStr=uint32  SampleTime=-1
  Constant8 : Constant  Value=212  OutDataTypeStr=uint32  SampleTime=-1
  Data Store Read45 : DataStoreRead  DataStoreName=oTilt  DataStoreElements=oTilt.oMot_.oIn_.fIPhaseMagnitude_  IndexOptions=Index vector (dialog)  Indices=1  OutputSizes=1
  Data Store Read79 : DataStoreRead  DataStoreName=oTilt  DataStoreElements=oTilt.oMot_.oState_.uiDriveState_  IndexOptions=Index vector (dialog)  Indices=1  OutputSizes=1
  Data Store Read81 : DataStoreRead  DataStoreName=oTilt  DataStoreElements=oTilt.oMot_.oParam_.fTripLimitSoftwareA_  IndexOptions=Index vector (dialog)  Indices=1  OutputSizes=1
  Equal1 : RelationalOperator  Operator===  OutDataTypeStr=boolean  RndMeth=Simplest
  Equal2 : RelationalOperator  Operator===  OutDataTypeStr=boolean  RndMeth=Simplest
  Forced_angle_overcurrent : Subsystem  TreatAsAtomicUnit=on
  GreaterThan3 : RelationalOperator  Operator=>  OutDataTypeStr=boolean  RndMeth=Simplest
  OR : Logic  Operator=OR  AllPortsSameDT=off  OutDataTypeStr=boolean
  checkForHwOvercurrents(&oTilt) : Subsystem  TreatAsAtomicUnit=on
  softwareOvercurrentProtection : Stateflow chart  TreatAsAtomicUnit=on
  wires:
  Constant8/1 -> Equal2/1
  Equal2/1 -> OR/1
  Equal1/1 -> OR/2
  OR/1 -> Forced_angle_overcurrent/Enable
  Data Store Read79/1 -> Equal1/1, Equal2/2
  Constant7/1 -> Equal1/2
  GreaterThan3/1 -> checkForHwOvercurrents(&oTilt)/Enable
  Data Store Read45/1 -> GreaterThan3/1
  Data Store Read81/1 -> GreaterThan3/2

== system Target_Control_System/Target_Control_System/Simulation Controls/Simulation Data Store Initialization/parameter_init_prop/initializeMotorTaskParameterPropulsion()/Sim Options Prop Forced Angle Variant Subsystem ==
  note: 1) Add Subsystem or Model blocks as valid variant choices.
      | 2) You cannot connect blocks at this level. At simulation, connectivity is automatically
      | determined, based on the active variant and port name matching.
  Sim Options 0 Prop Forced Angle Subsystem : Subsystem  VariantControl=(default)
  Sim Options 1 Prop Forced Angle Subsystem : Subsystem  VariantControl=SIMULATION_OPTIONS == 1 && TARGET_CODE_GEN ~= 1
  Out1 : Outport

== system Target_Control_System/Target_Control_System/Simulation Controls/Simulation Data Store Initialization/parameter_init_pump/initializeMotorTaskParameterPump()/Sim Options Pump Forced Angle Variant Subsystem ==
  note: 1) Add Subsystem or Model blocks as valid variant choices.
      | 2) You cannot connect blocks at this level. At simulation, connectivity is automatically
      | determined, based on the active variant and port name matching.
  Sim Options 0 Pump Forced Angle Subsystem : Subsystem  VariantControl=(default)
  Sim Options 1 Pump Forced Angle Subsystem : Subsystem  VariantControl=SIMULATION_OPTIONS == 1 && TARGET_CODE_GEN ~= 1
  Out1 : Outport

== system Target_Control_System/Target_Control_System/Simulation Controls/Simulation Data Store Initialization/setPositionControlModeTilt()/Enabled Subsystem/Switch Case Action Subsystem eNormal ==
  Action Port : ActionPort
  Constant : Constant  Value=0  OutDataTypeStr=single
  Constant1 : Constant  Value=0  OutDataTypeStr=single
  Constant2 : Constant  Value=0  OutDataTypeStr=single
  Data Store Write : DataStoreWrite  DataStoreName=oTilt  DataStoreElements=oTilt.oMot_.oParam_.oPid2DataRpmCtrl_.oParameter_.fIntegratorLeakFactor_  IndexOptions=Index vector (dialog)  Indices=1  OutputSizes=1
  Data Store Write1 : DataStoreWrite  DataStoreName=oTilt  DataStoreElements=oTilt.oMot_.oParam_.oPid2DataRpmCtrl_.oParameter_.fErrorReduction_  IndexOptions=Index vector (dialog)  Indices=1  OutputSizes=1
  Data Store Write2 : DataStoreWrite  DataStoreName=oTilt  DataStoreElements=oTilt.oMot_.oState_.oPosSensor_.oPidDataPosCtrl_.oParameter_.fErrorReduction_  IndexOptions=Index vector (dialog)  Indices=1  OutputSizes=1
  wires:
  Constant/1 -> Data Store Write/1
  Constant1/1 -> Data Store Write1/1
  Constant2/1 -> Data Store Write2/1

== system Target_Control_System/Target_Control_System/Simulation Controls/Simulation Data Store Initialization/setPositionControlModeTilt()/Enabled Subsystem/Switch Case Action Subsystem eNormalWithDeadZone ==
  Action Port : ActionPort
  Constant : Constant  Value=SLAVE_RPM_CTRL_INTEGRATOR_LEAKAGE_FACTOR__TILT  OutDataTypeStr=single
  Constant1 : Constant  Value=SLAVE_RPM_CTRL_ERROR_REDUCTION_RADS_PER_S__TILT  OutDataTypeStr=single
  Constant2 : Constant  Value=SLAVE_POS_CTRL_ERROR_REDUCTION_RAD__TILT  OutDataTypeStr=single
  Data Store Write : DataStoreWrite  DataStoreName=oTilt  DataStoreElements=oTilt.oMot_.oParam_.oPid2DataRpmCtrl_.oParameter_.fIntegratorLeakFactor_  IndexOptions=Index vector (dialog)  Indices=1  OutputSizes=1
  Data Store Write1 : DataStoreWrite  DataStoreName=oTilt  DataStoreElements=oTilt.oMot_.oParam_.oPid2DataRpmCtrl_.oParameter_.fErrorReduction_  IndexOptions=Index vector (dialog)  Indices=1  OutputSizes=1
  Data Store Write2 : DataStoreWrite  DataStoreName=oTilt  DataStoreElements=oTilt.oMot_.oState_.oPosSensor_.oPidDataPosCtrl_.oParameter_.fErrorReduction_  IndexOptions=Index vector (dialog)  Indices=1  OutputSizes=1
  wires:
  Constant2/1 -> Data Store Write2/1
  Constant1/1 -> Data Store Write1/1
  Constant/1 -> Data Store Write/1
